simulink model "Third_Model_2026_Dynamic_Target_Circ_Ship_WET"  (R2022b)
settings: Solver=VariableStepAuto  StartTime=0.0  StopTime=48  RelTol=1e-3
model workspace (MAT data in the model file):
  dt = 0.01
settings Model: Creator=user  LastModifiedBy=shova

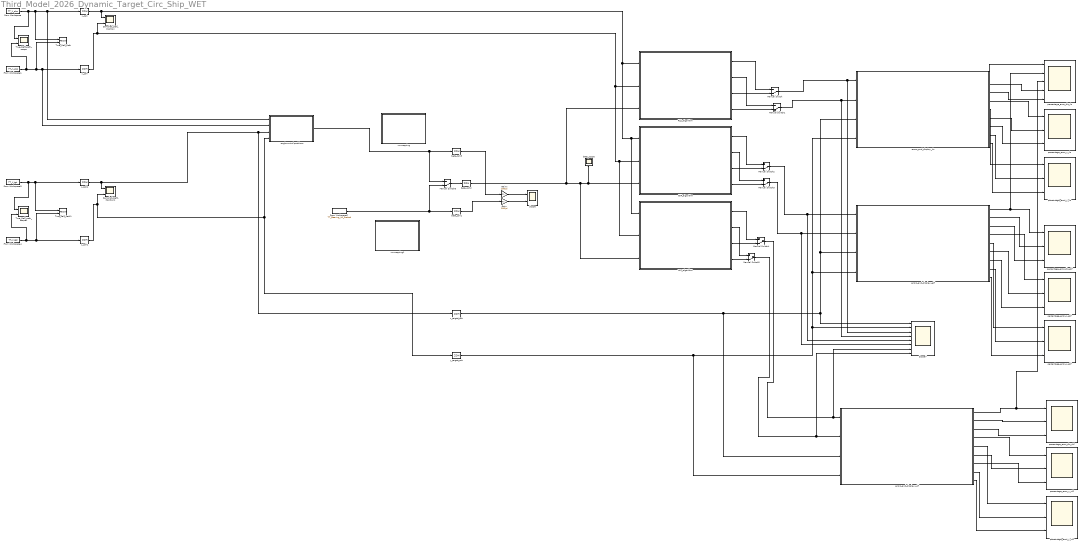
== system Third_Model_2026_Dynamic_Target_Circ_Ship_WET ==
  EKF_algorithm : Subsystem
  From Workspace : FromWorkspace  VariableName=TT_X_obs  SampleTime=1  OutputAfterFinalValue=Holding final value
  From Workspace1 : FromWorkspace  VariableName=TT_Y_obs  SampleTime=1  OutputAfterFinalValue=Holding final value
  From Workspace2 : FromWorkspace  VariableName=TT_Bearing_Inf_Scaled  SampleTime=1  OutputAfterFinalValue=Holding final value
  From Workspace3 : FromWorkspace  VariableName=TT_X_tgt  SampleTime=1  OutputAfterFinalValue=Holding final value
  From Workspace4 : FromWorkspace  VariableName=TT_Y_tgt  SampleTime=1  OutputAfterFinalValue=Holding final value
  Gain : Gain  Gain=180/pi
  Gain1 : Gain  Gain=180/pi
  Manual Switch{,1..6} (7 alike) : ManualSwitch  CurrentSetting=0
  RLS_algorithm : Subsystem
  Sampled_Self_Position : Scope  NumInputPorts=2
  Sampled_Self_Position1 : Scope  NumInputPorts=2
  Scope : Scope  NumInputPorts=2
  Scope7 : Scope  NumInputPorts=8
  True_Self_Path : Record  FileSettingsInternal="{\"entries\":[{\"content\":{\"excelSettings\":{\"content\":{},\"type\":\"Streamout.ExcelSettings\"}},\"type\":\"Streamout.FileSettingStorage\",\"uuid\":\"\"}],\"packageUris\":[\"http:\\/\\/schema.mathworks.com\\/mf0\\/streamout_blocks\\/R2020a\"],\"version\":\"1.0\"}"  Layout=[1 1]  SignalsInternal="{\"entries\":[{\"content\":{\"signals\":[{\"content\":{\"blockPath\":[],\"channel\":[],\"dimensions\":[1],\"domain\":\"\",\"lineColor\":\"#edb120\",\"plots\":[],\"port\":1,\"sid\":[\"\"],\"signalID\":3249,\"signalName\":\"From\\nWorkspace\"},\"type\":\"RecordBlkView.Signal\",\"uuid\":\"\"},{\"content\":{\"blockPath\":[],\"channel\":[],\"dimensions\":[1],\"domain\":\"\",\"lineColor\":\"#7e2f8e\",\"plots\":[],\"port\":2,\"sid\":[\"\"],\"signalID\":3253,\"signalName\":\"From\\nWorkspace1\"},\"type\":\"RecordBlkView.Signal\",\"uuid\":\"\"}]},\"type\":\"RecordBlkView.InputSignals\",\"uuid\":\"\"}],\"packageUris\":[\"http:\\/\\/schema.mathworks.com\\/mf0\\/streamout_blocks\\/R2020a\"],\"version\":\"1.0\"}"  VisualizationBindings="{\"xyplotplugin\":{\"info\":[{\"series\":[],\"subplotID\":1}]}}"  CompatibilityTag=XY
  True_Self_Path1 : Record  FileSettingsInternal="{\"entries\":[{\"content\":{\"excelSettings\":{\"content\":{},\"type\":\"Streamout.ExcelSettings\"}},\"type\":\"Streamout.FileSettingStorage\",\"uuid\":\"\"}],\"packageUris\":[\"http:\\/\\/schema.mathworks.com\\/mf0\\/streamout_blocks\\/R2020a\"],\"version\":\"1.0\"}"  Layout=[1 1]  SignalsInternal="{\"entries\":[{\"content\":{\"signals\":[{\"content\":{\"blockPath\":[],\"channel\":[],\"dimensions\":[1],\"domain\":\"\",\"lineColor\":\"#77ac30\",\"plots\":[],\"port\":1,\"sid\":[\"\"],\"signalID\":3257,\"signalName\":\"From\\nWorkspace3\"},\"type\":\"RecordBlkView.Signal\",\"uuid\":\"\"},{\"content\":{\"blockPath\":[],\"channel\":[],\"dimensions\":[1],\"domain\":\"\",\"lineColor\":\"#4dbeee\",\"plots\":[],\"port\":2,\"sid\":[\"\"],\"signalID\":3261,\"signalName\":\"From\\nWorkspace4\"},\"type\":\"RecordBlkView.Signal\",\"uuid\":\"\"}]},\"type\":\"RecordBlkView.InputSignals\",\"uuid\":\"\"}],\"packageUris\":[\"http:\\/\\/schema.mathworks.com\\/mf0\\/streamout_blocks\\/R2020a\"],\"version\":\"1.0\"}"  VisualizationBindings="{\"xyplotplugin\":{\"info\":[{\"series\":[],\"subplotID\":1}]}}"  CompatibilityTag=XY
  True_Self_path_scope : Scope  NumInputPorts=2
  True_Self_path_scope1 : Scope  NumInputPorts=2
  UKF_algorithm : Subsystem
  angle out of positions : MATLAB Function  TreatAsAtomicUnit=on
  beta_scope : Scope
  beta_zoh1 : ZeroOrderHold  SampleTime=dt
  beta_zoh2 : ZeroOrderHold  SampleTime=dt
  beta_zoh3 : ZeroOrderHold  SampleTime=dt
  errors_and_display_ekf : Subsystem
  errors_and_display_rls : Subsystem
  errors_and_display_ukf : Subsystem
  percentage_error_dis_ekf : Scope  NumInputPorts=3
  percentage_error_dis_rls : Scope  NumInputPorts=5
  percentage_error_dis_ukf : Scope  NumInputPorts=3
  percentage_error_x_ekf : Scope  NumInputPorts=3
  percentage_error_x_rls : Scope  NumInputPorts=3
  percentage_error_x_ukf : Scope  NumInputPorts=3
  percentage_error_y_ekf : Scope  NumInputPorts=3
  percentage_error_y_rls : Scope  NumInputPorts=3
  percentage_error_y_ukf : Scope  NumInputPorts=3
  unwrapping : MATLAB Function  TreatAsAtomicUnit=on
  unwrapping1 : MATLAB Function  TreatAsAtomicUnit=on
  x_target_zoh : ZeroOrderHold  SampleTime=dt
  x_zoh : ZeroOrderHold  SampleTime=dt
  x_zoh1 : ZeroOrderHold  SampleTime=dt
  y_target_zoh : ZeroOrderHold  SampleTime=dt
  y_zoh : ZeroOrderHold  SampleTime=dt
  y_zoh1 : ZeroOrderHold  SampleTime=dt
  wires:
  errors_and_display_rls/3(minus_ten_percentage_dis_target) -> percentage_error_dis_rls/5
  errors_and_display_ukf/6(ten_precentage_x_real) -> percentage_error_x_ukf/2
  From Workspace1/1 -> True_Self_Path/2, y_zoh/1, angle out of positions/2(self_pos_y), True_Self_path_scope/2
  y_target_zoh/1 -> errors_and_display_ekf/4(y_target), errors_and_display_rls/4(y_target), Scope7/2, errors_and_display_ukf/4(y_target)  "y_target"
  EKF_algorithm/3(x_ekf_dynamic) -> Manual Switch2/2
  Manual Switch5/1 -> Scope7/8, errors_and_display_ukf/2(y_ukf)
  x_zoh/1 -> Sampled_Self_Position/1, RLS_algorithm/1(x_i), UKF_algorithm/1(x_i), EKF_algorithm/1(x_i)
  errors_and_display_rls/4(percentage_error_x_rls) -> percentage_error_x_rls/1
  errors_and_display_rls/2(ten_percentage_dis_target) -> percentage_error_dis_rls/4
  errors_and_display_ekf/8(ten_precentage_y_real) -> percentage_error_y_ekf/2
  errors_and_display_rls/8(ten_precentage_y_real) -> percentage_error_y_rls/2
  errors_and_display_ekf/4(percentage_error_x_ekf) -> percentage_error_x_ekf/1
  errors_and_display_rls/1(percentage_error_dis_rls) -> percentage_error_dis_rls/1
  UKF_algorithm/2(y_ukf_static) -> Manual Switch5/1
  errors_and_display_ekf/5(percentage_error_y_ekf) -> percentage_error_y_ekf/1
  errors_and_display_ukf/3(minus_ten_percentage_dis_target) -> percentage_error_dis_ukf/3
  RLS_algorithm/3(x_rls_dynamic) -> Manual Switch/2
  errors_and_display_ekf/3(minus_ten_percentage_dis_target) -> percentage_error_dis_ekf/3
  EKF_algorithm/2(y_ekf_static) -> Manual Switch3/1
  RLS_algorithm/4(y_rls_dynamic) -> Manual Switch1/2
  y_zoh/1 -> Sampled_Self_Position/2, RLS_algorithm/2(y_i), UKF_algorithm/2(y_i), EKF_algorithm/2(y_i)
  errors_and_display_ukf/9(minus_ten_precentage_y_real) -> percentage_error_y_ukf/3
  beta_zoh2/1 -> RLS_algorithm/3(beta), UKF_algorithm/3(beta), beta_scope/1, EKF_algorithm/3(beta)
  beta_zoh3/1 -> Gain1/1
  From Workspace2/1 -> beta_zoh1/1, Manual Switch6/2
  UKF_algorithm/4(y_ukf_dynamic) -> Manual Switch5/2
  angle out of positions/1(beta) -> Manual Switch6/1, beta_zoh3/1
  Gain/1 -> Scope/2  "Measured"
  errors_and_display_ekf/6(ten_precentage_x_real) -> percentage_error_x_ekf/2
  RLS_algorithm/2(y_rls_static) -> Manual Switch1/1
  errors_and_display_ekf/1(percentage_error_dis_ekf) -> percentage_error_dis_rls/2, percentage_error_dis_ekf/1
  EKF_algorithm/1(x_ekf_static) -> Manual Switch2/1
  errors_and_display_ukf/5(percentage_error_y_ukf) -> percentage_error_y_ukf/1
  errors_and_display_ekf/2(ten_percentage_dis_target) -> percentage_error_dis_ekf/2
  errors_and_display_ekf/7(minus_ten_precentage_x_real) -> percentage_error_x_ekf/3
  x_target_zoh/1 -> errors_and_display_ekf/3(x_target), errors_and_display_rls/3(x_target), Scope7/1, errors_and_display_ukf/3(x_target)  "x_target"
  Manual Switch2/1 -> Scope7/5, errors_and_display_ekf/1(x_ekf)
  Gain1/1 -> Scope/1  "Theoretical"
  errors_and_display_ekf/9(minus_ten_precentage_y_real) -> percentage_error_y_ekf/3
  errors_and_display_ukf/2(ten_percentage_dis_target) -> percentage_error_dis_ukf/2
  Manual Switch3/1 -> Scope7/6, errors_and_display_ekf/2(y_ekf)
  errors_and_display_rls/9(minus_ten_precentage_y_real) -> percentage_error_y_rls/3
  beta_zoh1/1 -> Gain/1
  UKF_algorithm/1(x_ukf_static) -> Manual Switch4/1
  EKF_algorithm/4(y_ekf_dynamic) -> Manual Switch3/2
  errors_and_display_ukf/7(minus_ten_precentage_x_real) -> percentage_error_x_ukf/3
  RLS_algorithm/1(x_rls_static) -> Manual Switch/1
  errors_and_display_ukf/1(percentage_error_dis_ukf) -> percentage_error_dis_rls/3, percentage_error_dis_ukf/1
  Manual Switch1/1 -> Scope7/4, errors_and_display_rls/2(y_rls)
  From Workspace4/1 -> True_Self_Path1/2, y_zoh1/1, True_Self_path_scope1/2
  errors_and_display_ukf/8(ten_precentage_y_real) -> percentage_error_y_ukf/2
  From Workspace3/1 -> True_Self_path_scope1/1, True_Self_Path1/1, x_zoh1/1
  errors_and_display_rls/5(percentage_error_y_rls) -> percentage_error_y_rls/1
  Manual Switch6/1 -> beta_zoh2/1
  UKF_algorithm/3(x_ukf_dynamic) -> Manual Switch4/2
  y_zoh1/1 -> y_target_zoh/1, angle out of positions/4(target_pos_y), Sampled_Self_Position1/2
  errors_and_display_rls/7(minus_ten_precentage_x_real) -> percentage_error_x_rls/3
  errors_and_display_ukf/4(percentage_error_x_ukf) -> percentage_error_x_ukf/1
  Manual Switch4/1 -> Scope7/7, errors_and_display_ukf/1(x_ukf)
  Manual Switch/1 -> Scope7/3, errors_and_display_rls/1(x_rls)
  errors_and_display_rls/6(ten_precentage_x_real) -> percentage_error_x_rls/2
  From Workspace/1 -> True_Self_path_scope/1, True_Self_Path/1, x_zoh/1, angle out of positions/1(self_pos_x)
  x_zoh1/1 -> Sampled_Self_Position1/1, angle out of positions/3(target_pos_x), x_target_zoh/1

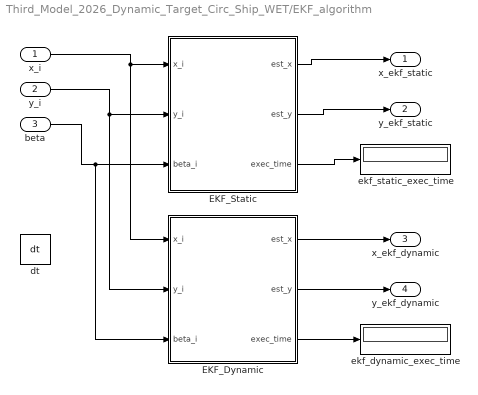
== system Third_Model_2026_Dynamic_Target_Circ_Ship_WET/EKF_algorithm ==
  x_i : Inport
  y_i : Inport  Port=2
  beta : Inport  Port=3
  EKF_Dynamic : MATLAB Function  TreatAsAtomicUnit=on
  EKF_Static : MATLAB Function  TreatAsAtomicUnit=on
  dt : Constant  Value=dt
  ekf_dynamic_exec_time : Display
      settings: Format=short_e
  ekf_static_exec_time : Display
      settings: Format=short_e
  x_ekf_static : Outport
  y_ekf_static : Outport  Port=2
  x_ekf_dynamic : Outport  Port=3
  y_ekf_dynamic : Outport  Port=4
  wires:
  x_i/1 -> EKF_Static/1(x_i), EKF_Dynamic/1(x_i)
  y_i/1 -> EKF_Dynamic/2(y_i), EKF_Static/2(y_i)
  beta/1 -> EKF_Static/3(beta_i), EKF_Dynamic/3(beta_i)
  EKF_Static/1(est_x) -> x_ekf_static/1
  EKF_Static/2(est_y) -> y_ekf_static/1
  EKF_Dynamic/1(est_x) -> x_ekf_dynamic/1
  EKF_Dynamic/2(est_y) -> y_ekf_dynamic/1
  EKF_Static/3(exec_time) -> ekf_static_exec_time/1
  EKF_Dynamic/3(exec_time) -> ekf_dynamic_exec_time/1

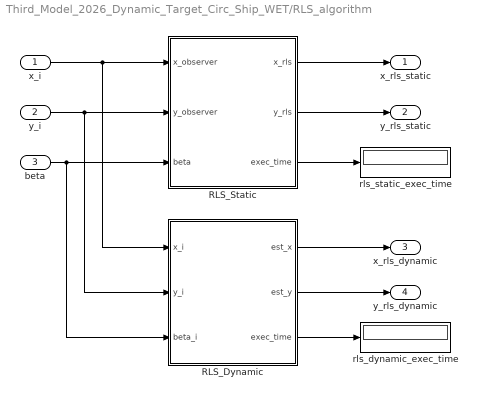
== system Third_Model_2026_Dynamic_Target_Circ_Ship_WET/RLS_algorithm ==
  x_i : Inport
  y_i : Inport  Port=2
  beta : Inport  Port=3
  RLS_Dynamic : MATLAB Function  TreatAsAtomicUnit=on
  RLS_Static : MATLAB Function  TreatAsAtomicUnit=on
  rls_dynamic_exec_time : Display
      settings: Format=short_e
  rls_static_exec_time : Display
      settings: Format=short_e
  x_rls_static : Outport
  y_rls_static : Outport  Port=2
  x_rls_dynamic : Outport  Port=3
  y_rls_dynamic : Outport  Port=4
  wires:
  x_i/1 -> RLS_Static/1(x_observer), RLS_Dynamic/1(x_i)
  y_i/1 -> RLS_Static/2(y_observer), RLS_Dynamic/2(y_i)
  beta/1 -> RLS_Static/3(beta), RLS_Dynamic/3(beta_i)
  RLS_Static/1(x_rls) -> x_rls_static/1
  RLS_Static/2(y_rls) -> y_rls_static/1
  RLS_Dynamic/1(est_x) -> x_rls_dynamic/1
  RLS_Dynamic/2(est_y) -> y_rls_dynamic/1
  RLS_Static/3(exec_time) -> rls_static_exec_time/1
  RLS_Dynamic/3(exec_time) -> rls_dynamic_exec_time/1

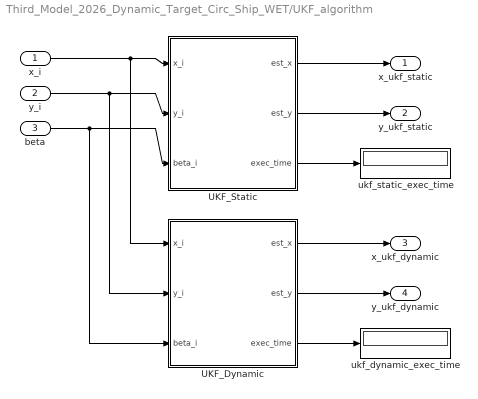
== system Third_Model_2026_Dynamic_Target_Circ_Ship_WET/UKF_algorithm ==
  x_i : Inport
  y_i : Inport  Port=2
  beta : Inport  Port=3
  UKF_Dynamic : MATLAB Function  TreatAsAtomicUnit=on
  UKF_Static : MATLAB Function  TreatAsAtomicUnit=on
  ukf_dynamic_exec_time : Display
      settings: Format=short_e
  ukf_static_exec_time : Display
      settings: Format=short_e
  x_ukf_static : Outport
  y_ukf_static : Outport  Port=2
  x_ukf_dynamic : Outport  Port=3
  y_ukf_dynamic : Outport  Port=4
  wires:
  x_i/1 -> UKF_Static/1(x_i), UKF_Dynamic/1(x_i)
  y_i/1 -> UKF_Dynamic/2(y_i), UKF_Static/2(y_i)
  beta/1 -> UKF_Static/3(beta_i), UKF_Dynamic/3(beta_i)
  UKF_Static/1(est_x) -> x_ukf_static/1
  UKF_Static/2(est_y) -> y_ukf_static/1
  UKF_Dynamic/1(est_x) -> x_ukf_dynamic/1
  UKF_Dynamic/2(est_y) -> y_ukf_dynamic/1
  UKF_Static/3(exec_time) -> ukf_static_exec_time/1
  UKF_Dynamic/3(exec_time) -> ukf_dynamic_exec_time/1

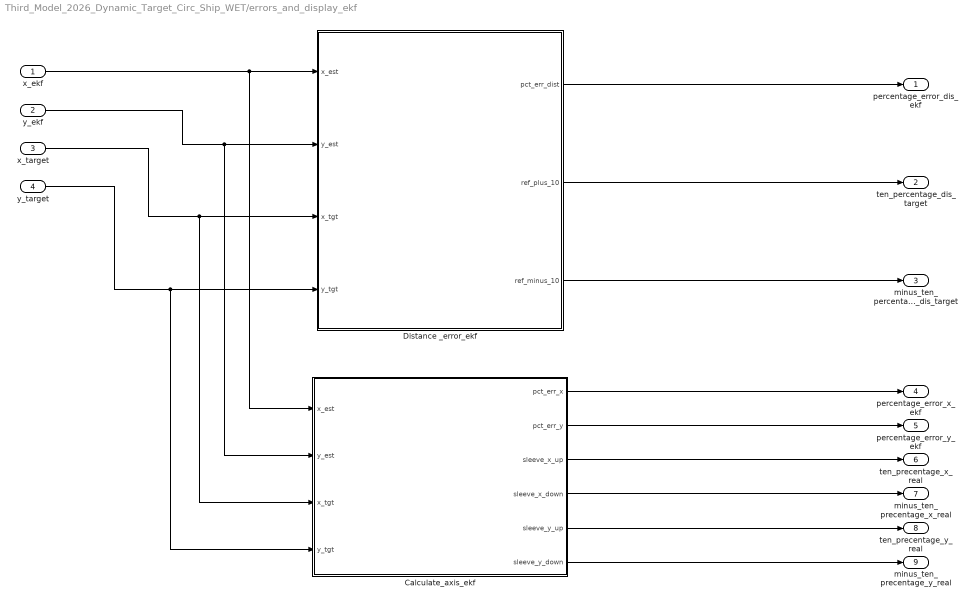
== system Third_Model_2026_Dynamic_Target_Circ_Ship_WET/errors_and_display_ekf ==
  x_ekf : Inport
  y_ekf : Inport  Port=2
  x_target : Inport  Port=3
  y_target : Inport  Port=4
  Calculate_axis_ekf : MATLAB Function  TreatAsAtomicUnit=on
  Distance _error_ekf : MATLAB Function  TreatAsAtomicUnit=on
  percentage_error_dis_ekf : Outport
  ten_percentage_dis_target : Outport  Port=2
  minus_ten_percentage_dis_target : Outport  Port=3
  percentage_error_x_ekf : Outport  Port=4
  percentage_error_y_ekf : Outport  Port=5
  ten_precentage_x_real : Outport  Port=6
  minus_ten_precentage_x_real : Outport  Port=7
  ten_precentage_y_real : Outport  Port=8
  minus_ten_precentage_y_real : Outport  Port=9
  wires:
  x_ekf/1 -> Distance _error_ekf/1(x_est), Calculate_axis_ekf/1(x_est)
  y_ekf/1 -> Distance _error_ekf/2(y_est), Calculate_axis_ekf/2(y_est)
  x_target/1 -> Distance _error_ekf/3(x_tgt), Calculate_axis_ekf/3(x_tgt)
  y_target/1 -> Calculate_axis_ekf/4(y_tgt), Distance _error_ekf/4(y_tgt)
  Distance _error_ekf/1(pct_err_dist) -> percentage_error_dis_ekf/1
  Distance _error_ekf/2(ref_plus_10) -> ten_percentage_dis_target/1
  Distance _error_ekf/3(ref_minus_10) -> minus_ten_percentage_dis_target/1
  Calculate_axis_ekf/1(pct_err_x) -> percentage_error_x_ekf/1
  Calculate_axis_ekf/2(pct_err_y) -> percentage_error_y_ekf/1
  Calculate_axis_ekf/3(sleeve_x_up) -> ten_precentage_x_real/1
  Calculate_axis_ekf/4(sleeve_x_down) -> minus_ten_precentage_x_real/1
  Calculate_axis_ekf/5(sleeve_y_up) -> ten_precentage_y_real/1
  Calculate_axis_ekf/6(sleeve_y_down) -> minus_ten_precentage_y_real/1

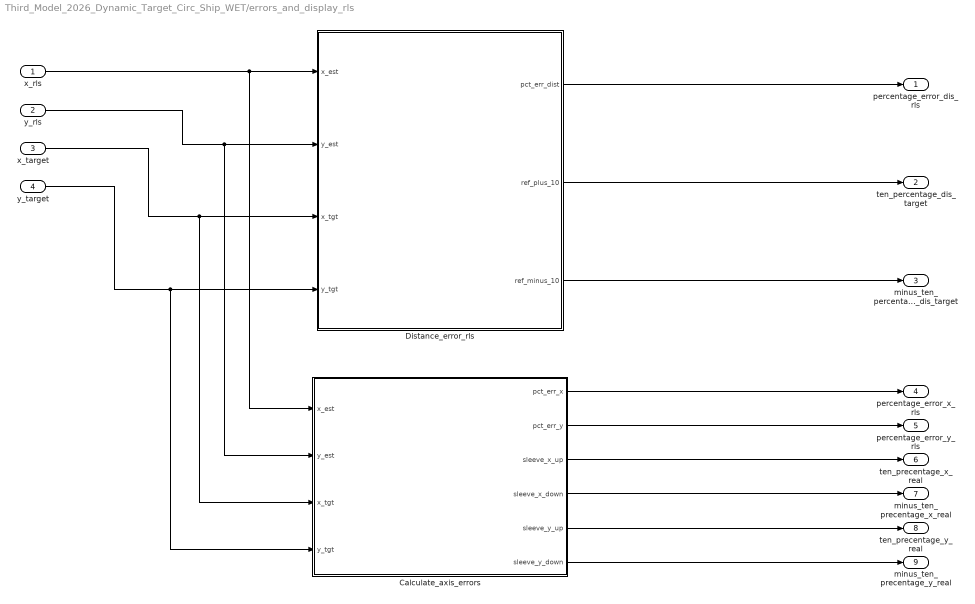
== system Third_Model_2026_Dynamic_Target_Circ_Ship_WET/errors_and_display_rls ==
  x_rls : Inport
  y_rls : Inport  Port=2
  x_target : Inport  Port=3
  y_target : Inport  Port=4
  Calculate_axis_errors : MATLAB Function  TreatAsAtomicUnit=on
  Distance_error_rls : MATLAB Function  TreatAsAtomicUnit=on
  percentage_error_dis_rls : Outport
  ten_percentage_dis_target : Outport  Port=2
  minus_ten_percentage_dis_target : Outport  Port=3
  percentage_error_x_rls : Outport  Port=4
  percentage_error_y_rls : Outport  Port=5
  ten_precentage_x_real : Outport  Port=6
  minus_ten_precentage_x_real : Outport  Port=7
  ten_precentage_y_real : Outport  Port=8
  minus_ten_precentage_y_real : Outport  Port=9
  wires:
  x_rls/1 -> Distance_error_rls/1(x_est), Calculate_axis_errors/1(x_est)
  y_rls/1 -> Distance_error_rls/2(y_est), Calculate_axis_errors/2(y_est)
  x_target/1 -> Distance_error_rls/3(x_tgt), Calculate_axis_errors/3(x_tgt)
  y_target/1 -> Calculate_axis_errors/4(y_tgt), Distance_error_rls/4(y_tgt)
  Distance_error_rls/1(pct_err_dist) -> percentage_error_dis_rls/1
  Distance_error_rls/2(ref_plus_10) -> ten_percentage_dis_target/1
  Distance_error_rls/3(ref_minus_10) -> minus_ten_percentage_dis_target/1
  Calculate_axis_errors/1(pct_err_x) -> percentage_error_x_rls/1
  Calculate_axis_errors/2(pct_err_y) -> percentage_error_y_rls/1
  Calculate_axis_errors/3(sleeve_x_up) -> ten_precentage_x_real/1
  Calculate_axis_errors/4(sleeve_x_down) -> minus_ten_precentage_x_real/1
  Calculate_axis_errors/5(sleeve_y_up) -> ten_precentage_y_real/1
  Calculate_axis_errors/6(sleeve_y_down) -> minus_ten_precentage_y_real/1

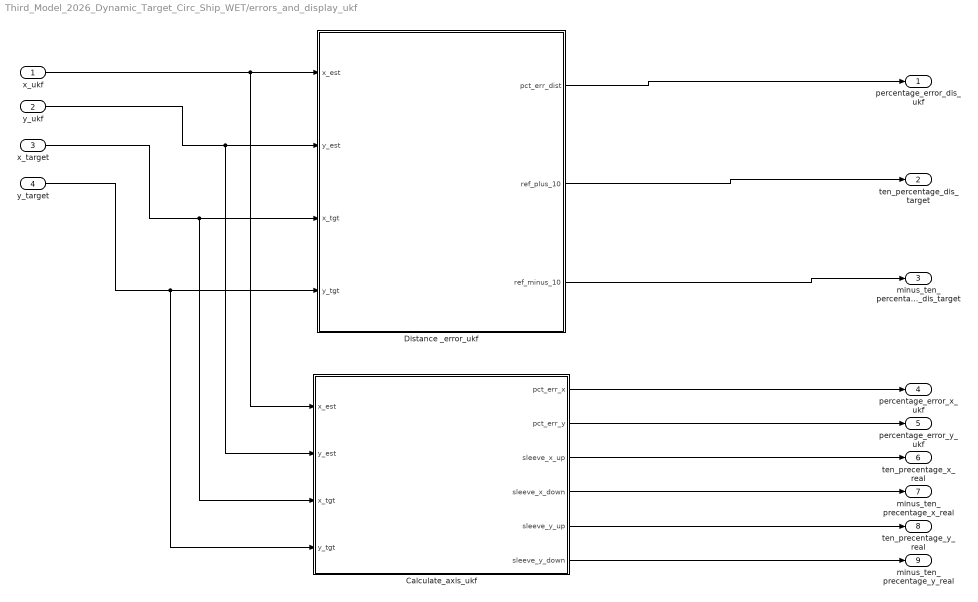
== system Third_Model_2026_Dynamic_Target_Circ_Ship_WET/errors_and_display_ukf ==
  x_ukf : Inport
  y_ukf : Inport  Port=2
  x_target : Inport  Port=3
  y_target : Inport  Port=4
  Calculate_axis_ukf : MATLAB Function  TreatAsAtomicUnit=on
  Distance _error_ukf : MATLAB Function  TreatAsAtomicUnit=on
  percentage_error_dis_ukf : Outport
  ten_percentage_dis_target : Outport  Port=2
  minus_ten_percentage_dis_target : Outport  Port=3
  percentage_error_x_ukf : Outport  Port=4
  percentage_error_y_ukf : Outport  Port=5
  ten_precentage_x_real : Outport  Port=6
  minus_ten_precentage_x_real : Outport  Port=7
  ten_precentage_y_real : Outport  Port=8
  minus_ten_precentage_y_real : Outport  Port=9
  wires:
  x_ukf/1 -> Distance _error_ukf/1(x_est), Calculate_axis_ukf/1(x_est)
  y_ukf/1 -> Distance _error_ukf/2(y_est), Calculate_axis_ukf/2(y_est)
  x_target/1 -> Distance _error_ukf/3(x_tgt), Calculate_axis_ukf/3(x_tgt)
  y_target/1 -> Calculate_axis_ukf/4(y_tgt), Distance _error_ukf/4(y_tgt)
  Distance _error_ukf/1(pct_err_dist) -> percentage_error_dis_ukf/1
  Distance _error_ukf/2(ref_plus_10) -> ten_percentage_dis_target/1
  Distance _error_ukf/3(ref_minus_10) -> minus_ten_percentage_dis_target/1
  Calculate_axis_ukf/1(pct_err_x) -> percentage_error_x_ukf/1
  Calculate_axis_ukf/2(pct_err_y) -> percentage_error_y_ukf/1
  Calculate_axis_ukf/3(sleeve_x_up) -> ten_precentage_x_real/1
  Calculate_axis_ukf/4(sleeve_x_down) -> minus_ten_precentage_x_real/1
  Calculate_axis_ukf/5(sleeve_y_up) -> ten_precentage_y_real/1
  Calculate_axis_ukf/6(sleeve_y_down) -> minus_ten_precentage_y_real/1

== matlab function Third_Model_2026_Dynamic_Target_Circ_Ship_WET/errors_and_display_ekf/Distance _error_ekf ==
  data: x_est input; pct_err_dist output; y_est input; x_tgt input; y_tgt input; ref_plus_10 output; ref_minus_10 output
function [pct_err_dist, ref_plus_10, ref_minus_10] = Distance_error_ekf(x_est, y_est, x_tgt, y_tgt)
    % Inputs:    % Inputs:
    %   x_est, y_est: Estimated position (from EKF)
    %   x_tgt, y_tgt: Real Target position
    
    % --- 1. Calculate Distances (Range) ---
    dist_est = sqrt(x_est^2 + y_est^2);
    dist_tgt = sqrt(x_tgt^2 + y_tgt^2);
    
    % Safety for division by zero
    if dist_tgt < 0.001
        dist_tgt = 0.001;
    end

    % --- 2. Calculate Percentage Error ---

    pos_err = sqrt((x_est - x_tgt)^2 + (y_est - y_tgt)^2);

    pct_err_dist = (pos_err / dist_tgt) * 100;
    
    % --- 3. Reference Lines (Constants) ---
    % Since the output is Percentage, the bounds are simply +10 and -10.
    ref_plus_10 = 10;
    ref_minus_10 = -10;
end

== matlab function Third_Model_2026_Dynamic_Target_Circ_Ship_WET/errors_and_display_ekf/Calculate_axis_ekf ==
  data: x_est input; pct_err_x output; y_est input; x_tgt input; y_tgt input; pct_err_y output; sleeve_x_up output; sleeve_x_down output; sleeve_y_up output; sleeve_y_down output
function [pct_err_x, pct_err_y, sleeve_x_up, sleeve_x_down, sleeve_y_up, sleeve_y_down] = Calculate_axis_errors(x_est, y_est, x_tgt, y_tgt)
    % Inputs:
    %   x_est, y_est: Estimated position
    %   x_tgt, y_tgt: Real Target position

    % --- 1. Calculate Percentage Errors (Per Axis) ---
    % Useful for statistics: "What is my % error on X?"
    if abs(x_tgt) < 0.001, x_tgt = 0.001; end
    if abs(y_tgt) < 0.001, y_tgt = 0.001; end
    
    pct_err_x = ((x_est - x_tgt) / x_tgt) * 100;
    pct_err_y = ((y_est - y_tgt) / y_tgt) * 100;

    % --- 2. Calculate Sleeve Bounds (The "Tunnel") ---
    % Useful for Visualization: Plot 'x_est' against these two lines.
    
    % Calculate 10% margin based on absolute position
    margin_x = 0.1 * abs(x_tgt);
    margin_y = 0.1 * abs(y_tgt);
    
    % Define Upper and Lower walls of the tunnel
    sleeve_x_up   = x_tgt + margin_x; % Real X + 10%
    sleeve_x_down = x_tgt - margin_x; % Real X - 10%
    
    sleeve_y_up   = y_tgt + margin_y; % Real Y + 10%
    sleeve_y_down = y_tgt - margin_y; % Real Y - 10%
end

== matlab function Third_Model_2026_Dynamic_Target_Circ_Ship_WET/UKF_algorithm/UKF_Dynamic ==
  data: x_i input; y_i input; beta_i input; est_x output; est_y output; exec_time output
function [est_x, est_y, exec_time] = UKF_Dynamic(x_i, y_i, beta_i)
    % UKF_Dynamic_Final (8-State)
    % Unscented Kalman Filter for Dynamic Target.
    % Jointly estimates Target (Pos+Vel) and Self (Pos+Vel).
    % State Vector: [Tx, Tvx, Ty, Tvy, Sx, Svx, Sy, Svy]
    
    persistent X_est P Q R 
    
    % --- Timing ---
    exec_time = 0; 
    coder.extrinsic('tic', 'toc'); 
    tStart = tic; 
    
    % --- Initialization (Runs once) ---
    if isempty(P)
        nx = 8; % 8 States
        
        % 1. Covariance (P)
        % High uncertainty (1000) to ensure fast convergence at start
        P = 10000 * eye(8); 
        
        % 2. Process Noise (Q) - 8x8 Matrix

        Q = 0.1 * diag([0.1, 0.01, 0.001, 0.001, 0.1, 0.001, 0.001, 0.01]);
        
        % 3. Measurement Noise (R) - 3x3 Matrix
        % [Var_Self_X, Var_Self_Y, Var_Constraint]
        % UPDATED based on your Simulink values:
        % - Self Position Noise = 5
        % - Constraint Noise = 1000 (Student value, kept as tuning parameter)
        R = diag([1, 1, 200]); 
    end
    
    if isempty(X_est)
        X_est = zeros(8, 1); 
    end
    
    % --- UKF Parameters (Calculated every step) ---
    nx = 8;
    alpha = 1e-3; 
    beta_param = 2; 
    kappa = 0; 
    lambda = alpha^2 * (nx + kappa) - nx;
    
    % Weights
    Wm = [lambda / (nx + lambda); repmat(1 / (2 * (nx + lambda)), 2 * nx, 1)];
    Wc = Wm;
    Wc(1) = Wc(1) + (1 - alpha^2 + beta_param);
    
    dt = 0.01; % Sample time (Match Simulink!)
    
    % ===========================================
    % 1. GENERATE SIGMA POINTS
    % ===========================================
    
    % FIX: Diagonal Loading (Replaces try/catch)
    % Ensures P is Positive Definite so chol() never crashes
    P_stable = P + 1e-9 * eye(nx);
    
    S = chol((nx + lambda) * P_stable, 'lower');
    sigma_points = [X_est, bsxfun(@plus, X_est, S), bsxfun(@minus, X_est, S)];
    
    % ===========================================
    % 2. PREDICT STEP (Time Update)
    % ===========================================
    
    % Pass through Dynamic Process Model (Constant Velocity)
    predicted_sigmas = process_model_dynamic(sigma_points, dt);
    
    % Recover Mean and Covariance
    [X_pred, P_pred] = compute_mean_and_cov(predicted_sigmas, Wm, Wc, Q);
    
    % ===========================================
    % 3. UPDATE STEP (Measurement Update)
    % ===========================================
    
    % Pass through Pseudolinear Measurement Model
    measured_sigmas = measurement_model(predicted_sigmas, beta_i);
    
    % Recover Measurement Mean and Covariance
    [y_pred, Pyy] = compute_mean_and_cov(measured_sigmas, Wm, Wc, R);
    
    % Cross-Covariance
    Pxy = compute_cross_cov(predicted_sigmas, measured_sigmas, X_pred, y_pred, Wc);
    
    % Kalman Gain
    K = Pxy / Pyy;
    
    % Measurement Vector
    z_meas = [x_i; y_i; 0]; 
    
    % Update State and Covariance
    resid = z_meas - y_pred;
    X_est = X_pred + K * resid;
    P = P_pred - K * Pyy * K';
    
    % Force Symmetry (Crucial for stability)
    P = 0.5 * (P + P');
    
    % --- Outputs ---
    est_x = X_est(1); % Target X
    est_y = X_est(3); % Target Y (Index 3 for 8-state vector!)
    
    exec_time = toc(tStart); 
end

%% --- Helper Functions ---

function points_out = process_model_dynamic(points_in, dt)
    % Dynamic Model (Constant Velocity for ALL 8 States)
    % x = x + vx*dt
    % vx = vx
    
    % The 8x8 Transition Matrix F
    F = [1 dt 0  0  0  0  0  0;  % Tx
         0  1 0  0  0  0  0  0;  % Tvx
         0  0 1 dt  0  0  0  0;  % Ty
         0  0 0  1  0  0  0  0;  % Tvy
         0  0 0  0  1 dt  0  0;  % Sx
         0  0 0  0  0  1  0  0;  % Svx
         0  0 0  0  0  0  1 dt;  % Sy
         0  0 0  0  0  0  0  1]; % Svy
         
    points_out = F * points_in;
end

function points_out = measurement_model(points_in, beta)
    % Pseudolinear Measurement Constraint
    % 0 = x_t*sin(b) - y_t*cos(b) - x_s*sin(b) + y_s*cos(b)
    
    s = sin(beta);
    c = cos(beta);
    
    % H Matrix (3x8)
    % Rows 1-2: Measure Self X (Idx 5) and Self Y (Idx 7)
    % Row 3: Constraint involving Tx(1), Ty(3), Sx(5), Sy(7)
    H = [0 0 0 0 1 0 0 0;
         0 0 0 0 0 0 1 0;
         s, 0, -c, 0, -s, 0, c, 0];
         
    points_out = H * points_in;
end

function [mean_out, cov_out] = compute_mean_and_cov(sigmas, Wm, Wc, NoiseCov)
    % Weighted Mean
    mean_out = sigmas * Wm;
    
    % Weighted Covariance
    d = bsxfun(@minus, sigmas, mean_out);
    cov_out = d * diag(Wc) * d' + NoiseCov;
end

function Pxy = compute_cross_cov(sig_pred, sig_meas, x_mean, y_mean, Wc)
    % Cross Covariance
    dx = bsxfun(@minus, sig_pred, x_mean);
    dy = bsxfun(@minus, sig_meas, y_mean);
    Pxy = dx * diag(Wc) * dy';
end

== matlab function Third_Model_2026_Dynamic_Target_Circ_Ship_WET/UKF_algorithm/UKF_Static ==
  data: x_i input; y_i input; beta_i input; est_x output; est_y output; exec_time output
function [est_x, est_y, exec_time] = UKF_Static(x_i, y_i, beta_i)
    % UKF_Static_Final
    % Unscented Kalman Filter for Static Target (6-State).
    % Estimates: [Target_X, Target_Y, Self_X, Self_Vx, Self_Y, Self_Vy]
    
    persistent X_est P Q R 
    
    % --- Timing ---
    exec_time = 0; 
    coder.extrinsic('tic', 'toc'); 
    tStart = tic; 
    
    % --- Initialization ---
    if isempty(P)
        nx = 6; % State Dimension
        
        % 1. Covariance (P) - High uncertainty
        P = 1000 * eye(nx); 
        
        % 2. Process Noise (Q)

        Q = 0.001 * diag([0.01, 0.01, 100, 10, 100, 10]); 
        
        % 3. Measurement Noise (R)
        % [Self_X, Self_Y, Constraint]
        % UPDATED: Matches your Simulink noise (5) and Constraint (200)
        R = diag([5, 5, 200]); 
    end
    
    if isempty(X_est)
        X_est = zeros(6, 1); 
    end
    
    % --- UKF Parameters (Calculated every step, like student code) ---
    nx = 6;
    alpha = 1e-3; 
    beta_param = 2; 
    kappa = 0; 
    lambda = alpha^2 * (nx + kappa) - nx;
    
    % Weights
    Wm = [lambda / (nx + lambda); repmat(1 / (2 * (nx + lambda)), 2 * nx, 1)];
    Wc = Wm;
    Wc(1) = Wc(1) + (1 - alpha^2 + beta_param);
    
    dt = 0.01; % Sample time
    
    % ===========================================
    % 1. GENERATE SIGMA POINTS
    % ===========================================
    
    % FIX: Diagonal Loading (Replaces try/catch)
    % Ensures P is Positive Definite so chol() never crashes
    P_stable = P + 1e-9 * eye(nx);
    
    S = chol((nx + lambda) * P_stable, 'lower');
    sigma_points = [X_est, bsxfun(@plus, X_est, S), bsxfun(@minus, X_est, S)];
    
    % ===========================================
    % 2. PREDICT STEP (Time Update)
    % ===========================================
    
    % Pass through Static Process Model (Target V=0)
    predicted_sigmas = process_model_static(sigma_points, dt);
    
    % Recover Mean and Covariance
    [X_pred, P_pred] = compute_mean_and_cov(predicted_sigmas, Wm, Wc, Q);
    
    % ===========================================
    % 3. UPDATE STEP (Measurement Update)
    % ===========================================
    
    % Pass through Pseudolinear Measurement Model
    measured_sigmas = measurement_model(predicted_sigmas, beta_i);
    
    % Recover Measurement Mean and Covariance
    [y_pred, Pyy] = compute_mean_and_cov(measured_sigmas, Wm, Wc, R);
    
    % Cross-Covariance
    Pxy = compute_cross_cov(predicted_sigmas, measured_sigmas, X_pred, y_pred, Wc);
    
    % Kalman Gain
    K = Pxy / Pyy;
    
    % Measurement Vector (Observed)
    z_meas = [x_i; y_i; 0]; 
    
    % Update State and Covariance
    resid = z_meas - y_pred;
    X_est = X_pred + K * resid;
    P = P_pred - K * Pyy * K';
    
    % SAFETY: Force Symmetry
    P = 0.5 * (P + P');
    
    % --- Outputs ---
    est_x = X_est(1); % Target X
    est_y = X_est(2); % Target Y
    
    exec_time = toc(tStart); 
end

%% --- Helper Functions ---

function points_out = process_model_static(points_in, dt)
    % Static Model: Target Velocity is 0. Self Velocity is constant.
    % 6x6 Matrix
    F = [1 0 0 0 0 0;  % Tx
         0 1 0 0 0 0;  % Ty
         0 0 1 dt 0 0; % Sx
         0 0 0 1 0 0;  % Svx
         0 0 0 0 1 dt; % Sy
         0 0 0 0 0 1]; % Svy
         
    points_out = F * points_in;
end

function points_out = measurement_model(points_in, beta)
    % Pseudolinear Measurement Matrix
    s = sin(beta);
    c = cos(beta);
    
    % H Matrix (3x6)
    % Rows 1-2: Measure Self X (Idx 3) and Self Y (Idx 5)
    % Row 3: Constraint involving Tx(1), Ty(2), Sx(3), Sy(5)
    H = [0 0 1 0 0 0;    % Self X
         0 0 0 0 1 0;    % Self Y
         s, -c, -s, 0, c, 0]; % Constraint
         
    points_out = H * points_in;
end

function [mean_out, cov_out] = compute_mean_and_cov(sigmas, Wm, Wc, NoiseCov)
    % Weighted Mean
    mean_out = sigmas * Wm;
    
    % Weighted Covariance
    d = bsxfun(@minus, sigmas, mean_out);
    cov_out = d * diag(Wc) * d' + NoiseCov;
end

function Pxy = compute_cross_cov(sig_pred, sig_meas, x_mean, y_mean, Wc)
    % Cross Covariance
    dx = bsxfun(@minus, sig_pred, x_mean);
    dy = bsxfun(@minus, sig_meas, y_mean);
    Pxy = dx * diag(Wc) * dy';
end

== matlab function Third_Model_2026_Dynamic_Target_Circ_Ship_WET/unwrapping1 ==
  settings: updateMethod=DISCRETE
  data: beta input; beta_unwrapped output
function beta_unwrapped = angle_unwrapper(beta)
%#codegen

% Persistent variable to store previous unwrapped angle
persistent beta_prev;
if isempty(beta_prev)
    beta_prev = 0;  % initial value on first call
end

% Define threshold for detecting 2π jumps
threshold = pi;

% Compute angle difference
delta = beta - mod(beta_prev, 2*pi);

% Unwrap: detect jumps larger than π and correct by ±2π
if delta > threshold
    delta = delta - 2*pi;
elseif delta < -threshold
    delta = delta + 2*pi;
end

% Update unwrapped angle
beta_unwrapped = beta_prev + delta;

% Save for next step
beta_prev = beta_unwrapped;

end

== matlab function Third_Model_2026_Dynamic_Target_Circ_Ship_WET/errors_and_display_ukf/Calculate_axis_ukf ==
  data: x_est input; pct_err_x output; y_est input; x_tgt input; y_tgt input; pct_err_y output; sleeve_x_up output; sleeve_x_down output; sleeve_y_up output; sleeve_y_down output
function [pct_err_x, pct_err_y, sleeve_x_up, sleeve_x_down, sleeve_y_up, sleeve_y_down] = Calculate_axis_errors(x_est, y_est, x_tgt, y_tgt)
    % Inputs:
    %   x_est, y_est: Estimated position
    %   x_tgt, y_tgt: Real Target position

    % --- 1. Calculate Percentage Errors (Per Axis) ---
    % Useful for statistics: "What is my % error on X?"
    if abs(x_tgt) < 0.001, x_tgt = 0.001; end
    if abs(y_tgt) < 0.001, y_tgt = 0.001; end
    
    pct_err_x = ((x_est - x_tgt) / x_tgt) * 100;
    pct_err_y = ((y_est - y_tgt) / y_tgt) * 100;

    % --- 2. Calculate Sleeve Bounds (The "Tunnel") ---
    % Useful for Visualization: Plot 'x_est' against these two lines.
    
    % Calculate 10% margin based on absolute position
    margin_x = 0.1 * abs(x_tgt);
    margin_y = 0.1 * abs(y_tgt);
    
    % Define Upper and Lower walls of the tunnel
    sleeve_x_up   = x_tgt + margin_x; % Real X + 10%
    sleeve_x_down = x_tgt - margin_x; % Real X - 10%
    
    sleeve_y_up   = y_tgt + margin_y; % Real Y + 10%
    sleeve_y_down = y_tgt - margin_y; % Real Y - 10%
end

== matlab function Third_Model_2026_Dynamic_Target_Circ_Ship_WET/errors_and_display_ukf/Distance _error_ukf ==
  data: x_est input; y_est input; pct_err_dist output; x_tgt input; y_tgt input; ref_plus_10 output; ref_minus_10 output
function [pct_err_dist, ref_plus_10, ref_minus_10] = Distance_error_ukf(x_est, y_est, x_tgt, y_tgt)
    % Inputs:
    %   x_est, y_est: Estimated position (from EKF)
    %   x_tgt, y_tgt: Real Target position
    
    % --- 1. Calculate Distances (Range) ---
    dist_est = sqrt(x_est^2 + y_est^2);
    dist_tgt = sqrt(x_tgt^2 + y_tgt^2);
    
    % Safety for division by zero
    if dist_tgt < 0.001
        dist_tgt = 0.001;
    end

    % --- 2. Calculate Percentage Error ---

    pos_err = sqrt((x_est - x_tgt)^2 + (y_est - y_tgt)^2);

    pct_err_dist = (pos_err / dist_tgt) * 100;
    
    % --- 3. Reference Lines (Constants) ---
    % Since the output is Percentage, the bounds are simply +10 and -10.
    ref_plus_10 = 10;
    ref_minus_10 = -10;
end

== matlab function Third_Model_2026_Dynamic_Target_Circ_Ship_WET/RLS_algorithm/RLS_Static ==
  data: x_observer input; y_observer input; beta input; x_rls output; y_rls output; exec_time output
function [x_rls, y_rls, exec_time] = RLS_Static(x_observer, y_observer, beta)
    % Inputs:
    %   x_observer, y_observer: Our ship's current position
    %   beta: Measured angle to target in radians

    persistent P X_est
    

    
    % Performance tracking
    exec_time = 0;
    coder.extrinsic('tic', 'toc');
    tStart = tic;

    % Initialization
    if isempty(P)
        P = 10000 * eye(2); % High initial uncertainty
        X_est = [0; 0];     % Initial guess (could be improved if you have a range guess)
    end

    % Pseudolinear Measurement Vector
    % Model: x_target * sin(beta) - y_target * cos(beta) = x_obs * sin(beta) - y_obs * cos(beta)
    
    sin_b = sin(beta);
    cos_b = cos(beta);

    % Measurement Matrix H
    H = [sin_b, -cos_b]; 
    
    % The "Pseudo-measurement" z
    z = x_observer * sin_b - y_observer * cos_b;

    % --- RLS Update ---
    
    % 1. Calculate Gain
    % We use R_cov here instead of '1'
    S = H * P * H' + 1; 
    K = (P * H') / S;

    % 2. Error (Innovation)
    e = z - H * X_est;

    % 3. Update State
    X_est = X_est + K * e;

    % 4. Update Covariance
    P = (eye(2) - K * H) * P;

    % --- Outputs ---
    x_rls = X_est(1);
    y_rls = X_est(2);
    exec_time = toc(tStart);
end

== matlab function Third_Model_2026_Dynamic_Target_Circ_Ship_WET/RLS_algorithm/RLS_Dynamic ==
  data: x_i input; y_i input; beta_i input; est_x output; est_y output; exec_time output
function [est_x, est_y, exec_time] = RLS_Dynamic(x_i, y_i, beta_i) 
% RLS_Dynamic_Final
% Performs Recursive Least Squares (RLS) tracking for a moving target.
% Inputs:
%
%   x_i, y_i : Our Ship's Position (Self)
%   beta_i   : Noisy Angle Measurement (Radians)
% Outputs:
%   est_x, est_y : Estimated Target Position

% --- Persistent Memory ---
persistent P X_i lambda lambda_rate

% --- Timing Setup ---
exec_time = 0; 
coder.extrinsic('tic', 'toc'); 
tStart = tic; 

% --- Initialization (Runs once at t=0) ---
if isempty(P)
    % We set P to 10000 so the filter isn't "stubborn" at the start.
    % It allows the estimate to snap to the true position in short time.
    P = 1000 * eye(2);  
    
    % FIX 2: Tuned Forgetting Factor (Lambda)
    % We start with a lower lambda to learn quickly, then slowly increase it.
    lambda = 0.6; 
    
    % The 'Rate' controls how fast it hardens. 
    lambda_rate = 0.996; 
end

if isempty(X_i)
    X_i = zeros(2, 1);  % X vector initialization as a zero vector
end

% --- 1. Construct Pseudolinear Measurement ---
% Measurement Vector (phi) and Scalar (z)
% Model: -x*sin(beta) + y*cos(beta) = y_obs*cos(beta) - x_obs*sin(beta)
phi_i = [-sin(beta_i); cos(beta_i)];
z_i   = y_i * cos(beta_i) - x_i * sin(beta_i);

% --- 2. Calculate RLS Updates ---

% A. Estimation Error
e = z_i - phi_i' * X_i;

% B. Calculate Gain Vector (g_k)
% We use 3e-5 for R (Noise Variance) to scale the denominator correctly.
R_cov = 3e-5; 
denominator = (lambda * R_cov) + (phi_i' * P * phi_i);
g_k = (P * phi_i) / denominator;

% C. Update State Vector (Position Estimate)
X_i = X_i + g_k * e;

% D. Update Covariance Matrix (P)
P = (1 / lambda) * (P - g_k * phi_i' * P);

% Prevents numerical crashes over long simulations.
P = 0.5 * (P + P');

% --- 3. Update Lambda (Annealing with Safety Cap) ---
% Slowly increase lambda to smooth out the noise...
lambda = lambda_rate * lambda + (1 - lambda_rate);

%if lambda > 0.9999999
%    lambda = 0.9999999;
%end

% --- Outputs ---
est_x = X_i(1);
est_y = X_i(2);
exec_time = toc(tStart); 
end

== matlab function Third_Model_2026_Dynamic_Target_Circ_Ship_WET/angle out of positions ==
  data: self_pos_x input; beta output; self_pos_y input; target_pos_x input; target_pos_y input
function beta = angle_beta_calc(self_pos_x, self_pos_y, target_pos_x, target_pos_y)

% Calculate relative position (target relative to self)
dx = target_pos_x - self_pos_x;   % delta x
dy = target_pos_y - self_pos_y;   % delta y

% Line-of-sight (bearing) angle beta from self to target
% atan2 returns angle in radians, from -pi to +pi
% Positive angle is counterclockwise from the positive x-axis
beta = atan2(dy, dx);

== matlab function Third_Model_2026_Dynamic_Target_Circ_Ship_WET/unwrapping ==
  settings: updateMethod=DISCRETE
  data: beta input; beta_unwrapped output
function beta_unwrapped = angle_unwrapper(beta)
%#codegen

% Persistent variable to store previous unwrapped angle
persistent beta_prev;
if isempty(beta_prev)
    beta_prev = 0;  % initial value on first call
end

% Define threshold for detecting 2π jumps
threshold = pi;

% Compute angle difference
delta = beta - mod(beta_prev, 2*pi);

% Unwrap: detect jumps larger than π and correct by ±2π
if delta > threshold
    delta = delta - 2*pi;
elseif delta < -threshold
    delta = delta + 2*pi;
end

% Update unwrapped angle
beta_unwrapped = beta_prev + delta;

% Save for next step
beta_prev = beta_unwrapped;

end

== matlab function Third_Model_2026_Dynamic_Target_Circ_Ship_WET/errors_and_display_rls/Distance_error_rls ==
  data: x_est input; pct_err_dist output; y_est input; x_tgt input; y_tgt input; ref_plus_10 output; ref_minus_10 output
function [pct_err_dist, ref_plus_10, ref_minus_10] = Distance_error_rls(x_est, y_est, x_tgt, y_tgt)
    % Inputs:
    %   x_est, y_est: Estimated position (from RLS)
    %   x_tgt, y_tgt: Real Target position
    
    % --- 1. Calculate Distances (Range) ---
    dist_est = sqrt(x_est^2 + y_est^2);
    dist_tgt = sqrt(x_tgt^2 + y_tgt^2);
    
    % Safety for division by zero
    if dist_tgt < 0.001
        dist_tgt = 0.001;
    end

    % --- 2. Calculate Percentage Error ---

    pos_err = sqrt((x_est - x_tgt)^2 + (y_est - y_tgt)^2);

    pct_err_dist = (pos_err / dist_tgt) * 100;
    
    % --- 3. Reference Lines (Constants) ---
    % Since the output is Percentage, the bounds are simply +10 and -10.
    ref_plus_10 = 10;
    ref_minus_10 = -10;
end

== matlab function Third_Model_2026_Dynamic_Target_Circ_Ship_WET/errors_and_display_rls/Calculate_axis_errors ==
  data: x_est input; pct_err_x output; y_est input; x_tgt input; y_tgt input; pct_err_y output; sleeve_x_up output; sleeve_x_down output; sleeve_y_up output; sleeve_y_down output
function [pct_err_x, pct_err_y, sleeve_x_up, sleeve_x_down, sleeve_y_up, sleeve_y_down] = Calculate_axis_errors(x_est, y_est, x_tgt, y_tgt)
    % Inputs:
    %   x_est, y_est: Estimated position
    %   x_tgt, y_tgt: Real Target position

    % --- 1. Calculate Percentage Errors (Per Axis) ---
    % Useful for statistics: "What is my % error on X?"
    if abs(x_tgt) < 0.001, x_tgt = 0.001; end
    if abs(y_tgt) < 0.001, y_tgt = 0.001; end
    
    pct_err_x = ((x_est - x_tgt) / x_tgt) * 100;
    pct_err_y = ((y_est - y_tgt) / y_tgt) * 100;

    % --- 2. Calculate Sleeve Bounds (The "Tunnel") ---
    % Useful for Visualization: Plot 'x_est' against these two lines.
    
    % Calculate 10% margin based on absolute position
    margin_x = 0.1 * abs(x_tgt);
    margin_y = 0.1 * abs(y_tgt);
    
    % Define Upper and Lower walls of the tunnel
    sleeve_x_up   = x_tgt + margin_x; % Real X + 10%
    sleeve_x_down = x_tgt - margin_x; % Real X - 10%
    
    sleeve_y_up   = y_tgt + margin_y; % Real Y + 10%
    sleeve_y_down = y_tgt - margin_y; % Real Y - 10%
end

== matlab function Third_Model_2026_Dynamic_Target_Circ_Ship_WET/EKF_algorithm/EKF_Dynamic ==
  data: x_i input; y_i input; beta_i input; est_x output; est_y output; exec_time output
function [est_x, est_y, exec_time] = EKF_Dynamic(x_i, y_i, beta_i)
    % EKF_Dynamic_StudentVersion (8-State)
    % Jointly estimates Target State (Pos+Vel) and Self State (Pos+Vel).

    
    persistent X_est P Q R
    
    % --- Timing ---
    exec_time = 0; 
    coder.extrinsic('tic', 'toc'); 
    tStart = tic;

    % --- Initialization ---
    if isempty(P)
        % 1. Covariance (P)
        % Start high (1000) so the filter doesn't stick to zero initially.
        % 1000 ensures faster convergence.
        P = 10000 * eye(8); 
        
        % 2. Process Noise (Q) - 8x8 Matrix

        Q = 0.1 * diag([0.1, 0.01, 0.001, 0.001, 0.1, 0.001, 0.001, 0.01]);
        
        % 3. Measurement Noise (R) - 3x3 Matrix
        % [Var_Self_X, Var_Self_Y, Var_Constraint]
        % UPDATED based on your Simulink values:
        % - Self Position Noise = 5
        % - Constraint Noise = 1000 (Student value, kept as tuning parameter)
        R = diag([1, 1, 200]); 
    end
    
    if isempty(X_est)
        X_est = zeros(8, 1); % [x_t; vx_t; y_t; vy_t; x_s; vx_s; y_s; vy_s]
    end

    % --- Constants ---
    dt = 0.01; % Sample Time 

    % --- 1. PREDICT STEP (Process Model) ---
    % Constant Velocity Model for ALL 8 states.
    % F matrix propagates position: x = x + vx*dt
    
    F = [1 dt 0  0  0  0  0  0;  % Target X
         0  1 0  0  0  0  0  0;  % Target Vx
         0  0 1 dt  0  0  0  0;  % Target Y
         0  0 0  1  0  0  0  0;  % Target Vy
         0  0 0  0  1 dt  0  0;  % Self X
         0  0 0  0  0  1  0  0;  % Self Vx
         0  0 0  0  0  0  1 dt;  % Self Y
         0  0 0  0  0  0  0  1]; % Self Vy
         
    % Predict State
    X_est = F * X_est;
    
    % Predict Covariance
    P = F * P * F' + Q;

    % --- 2. UPDATE STEP (Measurement) ---
    
    % Measurement Matrix (H) - 3x8
    % Rows 1-2: Measure Self Position (States 5 and 7)
    % Row 3: Pseudolinear Constraint: 0 = x_t*sin - y_t*cos - x_s*sin + y_s*cos
    
    sin_b = sin(beta_i);
    cos_b = cos(beta_i);
    
    % Note indices carefully:
    % Target X (1), Target Y (3) -> In constraint
    % Self X (5),   Self Y (7)   -> Measured directly & in constraint
    
    H = [0 0 0 0 1 0 0 0;  % Measure Self X (State 5)
         0 0 0 0 0 0 1 0;  % Measure Self Y (State 7)
         sin_b, 0, -cos_b, 0, -sin_b, 0, cos_b, 0]; % Constraint
         
    % Measurement Vector
    z_meas = [x_i; y_i; 0];
    
    % Residual
    y_hat = H * X_est;
    resid = z_meas - y_hat;
    
    % Kalman Gain
    S = H * P * H' + R;
    K = P * H' / S;
    
    % Update State
    X_est = X_est + K * resid;
    
    % Update Covariance
    P = (eye(8) - K * H) * P;
    
    % SAFETY: Force Symmetry (Prevents crashes in long simulations)
    P = 0.5 * (P + P');

    % --- Output ---
    est_x = X_est(1); % Target X
    est_y = X_est(3); % Target Y (Note: index 3, not 2!)
    
    exec_time = toc(tStart); 
end

== matlab function Third_Model_2026_Dynamic_Target_Circ_Ship_WET/EKF_algorithm/EKF_Static ==
  data: x_i input; y_i input; est_x output; est_y output; exec_time output; beta_i input
function [est_x, est_y, exec_time] = EKF_Static(x_i, y_i, beta_i)
    % EKF_Static_StudentVersion
    % Implementation of the 6-State Pseudolinear EKF (Joint Estimation).
    % Estimates both Target Position and Own-Ship State.
    
    persistent X_est P Q R
    
    % --- Timing ---
    exec_time = 0; 
    coder.extrinsic('tic', 'toc'); 
    tStart = tic;
    
    % --- Initialization ---
    if isempty(P)
        % 1. Covariance (P)
        % High uncertainty (1000) for all 6 states
        P = 1000 * eye(6); 
        
        % 2. Process Noise (Q)
        % Matches the student document:
        % [x_t, y_t, x_i, vx_i, y_i, vy_i]
        % Low noise for target (static), Higher for self-ship (dynamic)
        Q = 0.001 * diag([0.01, 0.01, 100, 10, 100, 10]); 
        
        % 3. Measurement Noise (R)
        % [x_self_meas; y_self_meas; pseudo_residual]
        % Note: The 3rd value (200) is the noise variance for the angle constraint
        R = diag([5, 5, 200]); 
    end
    
    if isempty(X_est)
        % Initialize State: 6x1 Vector
        X_est = zeros(6, 1); 
    end
    
    % --- Constants ---
    dt = 0.01; 

    % --- 1. PREDICT STEP ---
    
    % Transition Matrix (F)
    % Target is static (Identity), Self is Constant Velocity (1, dt)
    F = [1 0 0 0 0 0;  % Target x
         0 1 0 0 0 0;  % Target y
         0 0 1 dt 0 0; % Self x
         0 0 0 1 0 0;  % Self vx
         0 0 0 0 1 dt; % Self y
         0 0 0 0 0 1]; % Self vy
         
    % Predict State
    X_est = F * X_est;
    
    % Predict Covariance
    P = F * P * F' + Q;
    
    % --- 2. UPDATE STEP ---
    
    % Measurement Matrix (H) - The Pseudolinear Form
    sin_b = sin(beta_i);
    cos_b = cos(beta_i);
    
    % Rows 1&2: Direct measurement of Own-Ship (x_i, y_i)
    % Row 3:   The Pseudo-Constraint (0 = x_t*sin - y_t*cos - x_i*sin + y_i*cos)
    H = [0 0 1 0 0 0;
         0 0 0 0 1 0;
         sin_b, -cos_b, -sin_b, 0, cos_b, 0];
         
    % Construct Measurement Vector (z)
    % We measure our own X, our own Y, and "0" for the constraint
    z_meas = [x_i; y_i; 0];
    
    % Calculate Residual (Innovation)
    y_hat = H * X_est;
    resid = z_meas - y_hat;
    
    % Kalman Gain
    S = H * P * H' + R;
    K = P * H' / S;
    
    % Update State
    X_est = X_est + K * resid;
    
    % Update Covariance
    P = (eye(6) - K * H) * P;
    
    % --- SAFETY FIX: Symmetry ---
    % It is REQUIRED to prevent crashes in long simulations (60s+).
    P = 0.5 * (P + P');

    % --- Output ---
    est_x = X_est(1); % Target X is state 1
    est_y = X_est(2); % Target Y is state 2
    
    exec_time = toc(tStart); 
end
